simulink model "AutomatiqueCoursSimuL2"  (R2024a)
settings: Solver=VariableStepAuto  StartTime=0.0  StopTime=10.0  RelTol=1e-3
values from neighbouring files (symbols this model uses):
  L = 0.2    [AutomatiqueCours.m]
  theta0 = asin( pi / 8)    [AutomatiqueCours.m]
libraries: eeStairGenerator x2
settings Model: Creator=cuvilli13u  LastModifiedBy=cuvilli13u

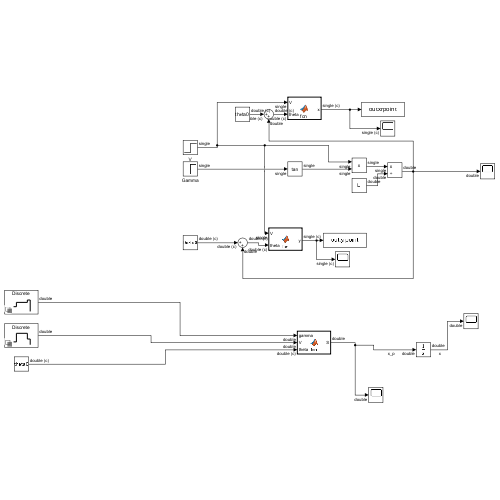
[thumbnail: Simulink's stored preview of the top-level diagram]
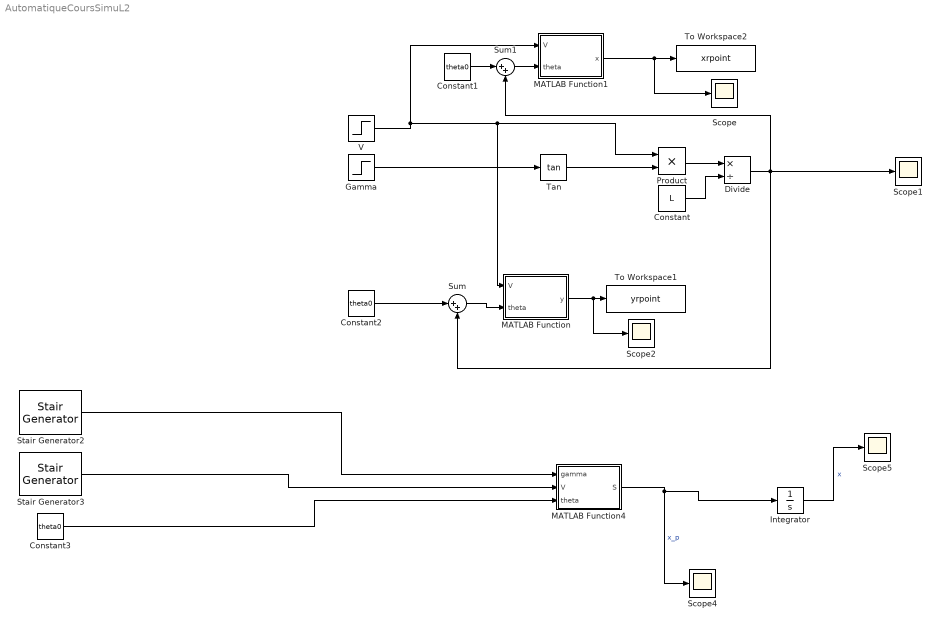
== system AutomatiqueCoursSimuL2 ==
  Constant : Constant  Value=L
  Constant1 : Constant  Value=theta0
  Constant2 : Constant  Value=theta0
  Constant3 : Constant  Value=theta0
  Divide : Product  Inputs=*/
  Gamma : Step  After=0.2  OutDataTypeStr=single  SampleTime=0
  Integrator : Integrator
  MATLAB Function : MATLAB Function  TreatAsAtomicUnit=on
  MATLAB Function1 : MATLAB Function  TreatAsAtomicUnit=on
  MATLAB Function4 : MATLAB Function  TreatAsAtomicUnit=on
  Product : Product
  Scope{,1..2,4..5} (5 alike) : Scope
  Stair Generator2 : eeStairGenerator/Stair Generator  LabelModeActiveChoice=Discrete  TimeInput=[0.5 1 3 3.5]  AmplitudeInput=[1 2 2.5 0]  SampleTime=-1  RepeatPattern=off  OutDataTypeStr=double
      settings: LibrarySourceBlock=ee_sl_lib/General Control/Stair Generator
  Stair Generator3 : eeStairGenerator/Stair Generator  LabelModeActiveChoice=Discrete  TimeInput=[0.5 1 3 3.5]  AmplitudeInput=[0.2 0.8 0.4 0]  SampleTime=-1  RepeatPattern=off  OutDataTypeStr=double
      settings: LibrarySourceBlock=ee_sl_lib/General Control/Stair Generator
  Sum : Sum  Inputs=|++
  Sum1 : Sum  Inputs=|++
  Tan : Trigonometry  Operator=tan
  To Workspace1 : ToWorkspace  VariableName=yrpoint  SampleTime=-1
  To Workspace2 : ToWorkspace  VariableName=xrpoint  SampleTime=-1
  V : Step  OutDataTypeStr=single  SampleTime=0
  wires:
  Gamma/1 -> Tan/1
  Tan/1 -> Product/2
  V/1 -> MATLAB Function/1(V), Product/1, MATLAB Function1/1(V)
  Product/1 -> Divide/1
  Constant/1 -> Divide/2
  Constant2/1 -> Sum/1
  Divide/1 -> Sum1/2, Scope1/1, Sum/2
  Sum/1 -> MATLAB Function/2(theta)
  MATLAB Function/1(y) -> Scope2/1, To Workspace1/1
  MATLAB Function1/1(x) -> Scope/1, To Workspace2/1
  Sum1/1 -> MATLAB Function1/2(theta)
  Constant1/1 -> Sum1/1
  Integrator/1 -> Scope5/1  "x"
  MATLAB Function4/1(S) -> Scope4/1, Integrator/1  "x_p"
  Stair Generator2/1 -> MATLAB Function4/1(gamma)
  Stair Generator3/1 -> MATLAB Function4/2(V)
  Constant3/1 -> MATLAB Function4/3(theta)

== matlab function AutomatiqueCoursSimuL2/MATLAB Function1 ==
  data: x output; V input; theta input
function x = fcn(V,theta)

x = V*cos(theta);

== matlab function AutomatiqueCoursSimuL2/MATLAB Function ==
  data: y output; V input; theta input
function y = fcn(V,theta)

y = V*sin(theta);

== matlab function AutomatiqueCoursSimuL2/MATLAB Function4 ==
  data: gamma input; S output; V input; theta input
function S = fcn(gamma, V,theta)

L=0.2;

xr      = V*cos(theta);
yr      = V*sin(theta);
thetap  = V*tan(gamma)/L


rho     =sqrt(xr^2 + yr^2)
alpha   = atan(yr/xr) - theta
% beta  = -1*alpha - thetar

rhop    = -V*cos(alpha)
alphap  = V*(sin(alpha)/rho - tan(gamma)/L)
betap   = -V*sin(alpha)/rho

S       = [xr ,yr ,thetap ,rhop ,alphap ,betap];
